simulink model "enable_held_with_pre"  (R2016a)
settings: Solver=VariableStepAuto  StartTime=0.0  StopTime=10.0  RelTol=1e-3
settings Model: Creator=hamza  LastModifiedBy=hamza

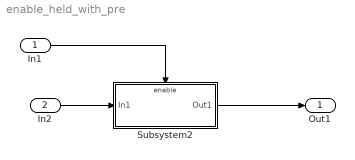
== system enable_held_with_pre ==
  In1 : Inport  OutDataTypeStr=boolean
  In2 : Inport  Port=2  OutDataTypeStr=double
  Subsystem2 : Subsystem  TreatAsAtomicUnit=on
  Out1 : Outport
  wires:
  In1/1 -> Subsystem2/Enable
  In2/1 -> Subsystem2/1(In1)
  Subsystem2/1(Out1) -> Out1/1

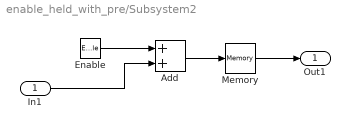
== system enable_held_with_pre/Subsystem2 ==
  In1 : Inport
  Enable : EnablePort  ShowOutputPort=on
  Add : Sum
  Memory : Memory
  Out1 : Outport
  wires:
  Enable/1 -> Add/1
  In1/1 -> Add/2
  Add/1 -> Memory/1
  Memory/1 -> Out1/1
